simulink model "Subsystem_qd_model"  (R2021a)
settings: Solver=VariableStepAuto  StartTime=0.0  StopTime=10.0  RelTol=1e-3
undefined symbols (not defined in the file): Dm, J, Lam, Lss, P, rs, Ts
settings Model: Creator=Utkarsh Anand  LastModifiedBy=Utkarsh Anand
settings DataIOCC: SaveOutput=off  SaveTime=off

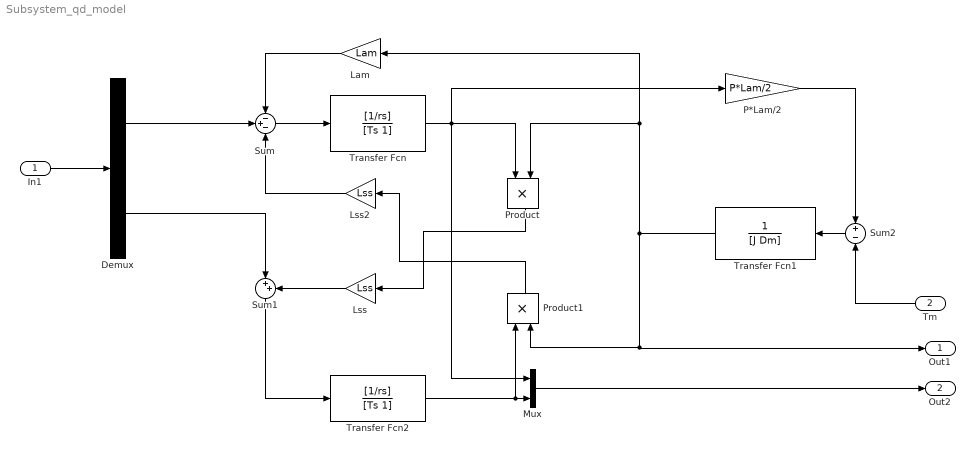
== system Subsystem_qd_model ==
  In1 : Inport  OutDataTypeStr=double  PortDimensions=2  SampleTime=0
  Tm : Inport  Port=2  OutDataTypeStr=double  PortDimensions=1  SampleTime=0
  Demux : Demux  Outputs=2
  Lam : Gain  Gain=Lam
  Lss : Gain  Gain=Lss
  Lss2 : Gain  Gain=Lss
  Mux : Mux  Inputs=2
  P*Lam/2 : Gain  Gain=P*Lam/2
  Product : Product
  Product1 : Product
  Sum : Sum  Inputs=-+-
  Sum1 : Sum  Inputs=|++
  Sum2 : Sum  Inputs=+-
  Transfer Fcn : TransferFcn  Numerator=[1/rs]  Denominator=[Ts 1]
  Transfer Fcn1 : TransferFcn  Denominator=[J Dm]
  Transfer Fcn2 : TransferFcn  Numerator=[1/rs]  Denominator=[Ts 1]
  Out1 : Outport  OutDataTypeStr=double  PortDimensions=1  SampleTime=0
  Out2 : Outport  Port=2  OutDataTypeStr=double  PortDimensions=2  SampleTime=0
  wires:
  Transfer Fcn2/1 -> Mux/2, Product1/1
  Mux/1 -> Out2/1
  P*Lam/2/1 -> Sum2/1
  Transfer Fcn/1 -> P*Lam/2/1, Product/1, Mux/1
  In1/1 -> Demux/1
  Transfer Fcn1/1 -> Product1/2, Out1/1, Lam/1, Product/2
  Sum1/1 -> Transfer Fcn2/1
  Lss2/1 -> Sum/3
  Sum/1 -> Transfer Fcn/1
  Lss/1 -> Sum1/2
  Sum2/1 -> Transfer Fcn1/1
  Product/1 -> Lss/1
  Product1/1 -> Lss2/1
  Lam/1 -> Sum/1
  Demux/1 -> Sum/2
  Demux/2 -> Sum1/1
  Tm/1 -> Sum2/2
